simulink model "moyenneur_ordre_2"  (R2019a)
settings: Solver=VariableStepAuto  StartTime=0.0  StopTime=10.0  RelTol=1e-3
libraries: Librairie x2
settings Model: Creator=shse  LastModifiedBy=shse

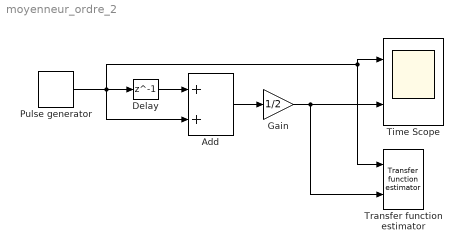
== system moyenneur_ordre_2 ==
  Add : Sum
  Delay : Delay  DelayLength=1  InitialCondition=0  InputProcessing=Columns as channels (frame based)
  Gain : Gain  Gain=1/2
  Pulse generator : Librairie/Pulse generator  fee=11025  NN=1024
  Time Scope : Scope  NumInputPorts=2
  Transfer function estimator : Librairie/Transfer function estimator  fee=11025  NN=1024
  wires:
  Gain/1 -> Transfer function estimator/2, Time Scope/2
  Add/1 -> Gain/1
  Delay/1 -> Add/1
  Pulse generator/1 -> Add/2, Transfer function estimator/1, Time Scope/1, Delay/1
